simulink model "multiFeedModel"  (R2022a)
settings: Solver=VariableStepAuto  StartTime=0.0  StopTime=168  RelTol=1e-3
model workspace (MAT data in the model file):
  Q_in = [0.12271780758; 0.123470790595; 0.124228393831; 0.124990645638; 0.125757574538; 0.12652920923; 0.127305578587]
libraries: simulink x1
settings Model: Creator=tomok  LastModifiedBy=tomok

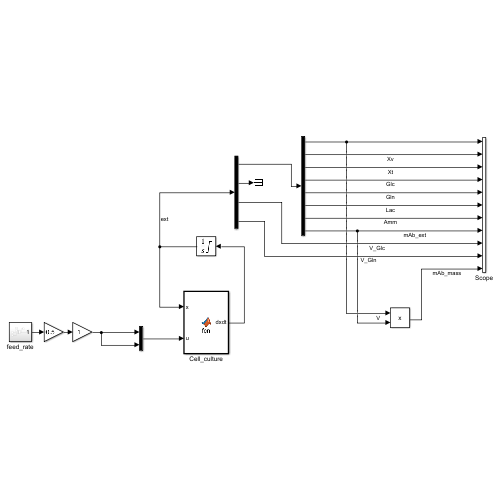
[thumbnail: Simulink's stored preview of the top-level diagram]
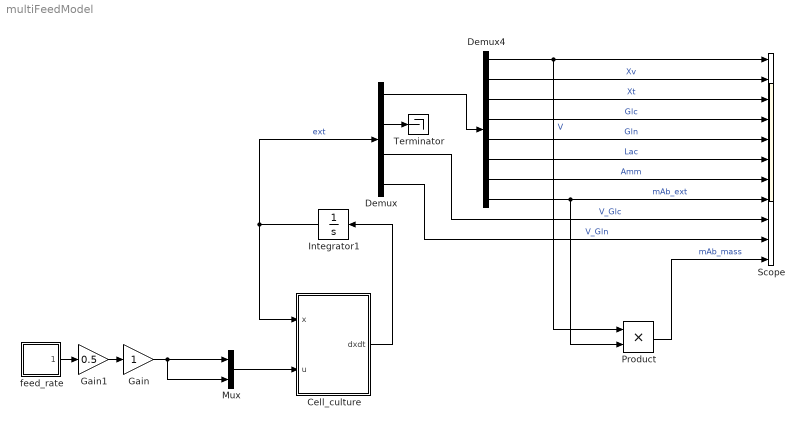
== system multiFeedModel ==
  Cell_culture : MATLAB Function  TreatAsAtomicUnit=on
  Demux : Demux  Outputs=[8,8,1,1]
  Demux4 : Demux  Outputs=8
  Gain : Gain
  Gain1 : Gain  Gain=0.5
  Integrator1 : Integrator  InitialCondition=|  LimitOutput=on  LowerSaturationLimit=0
      | [0.2; 2E+8;
      | 2E+8;
      | 25.1;
      | 5.01;
      | 0;
      | 0;
      | 100; zeros(8,1); 0; 0]
  Mux : Mux  Inputs=2
  Product : Product
  Scope : Scope  NumInputPorts=11
  Terminator : Terminator
  feed_rate : Subsystem
  wires:
  Demux4/1 -> Scope/1, Product/1  "V"
  Product/1 -> Scope/11  "mAb_mass"
  Mux/1 -> Cell_culture/2(u)
  Demux4/5 -> Scope/5  "Gln"
  Demux4/2 -> Scope/2  "Xv"
  Integrator1/1 -> Demux/1, Cell_culture/1(x)  "ext"
  Cell_culture/1(dxdt) -> Integrator1/1
  Demux4/3 -> Scope/3  "Xt"
  Demux4/4 -> Scope/4  "Glc"
  Demux4/7 -> Scope/7  "Amm"
  Demux4/6 -> Scope/6  "Lac"
  Demux4/8 -> Product/2, Scope/8  "mAb_ext"
  feed_rate/1(Out1) -> Gain1/1
  Gain/1 -> Mux/2, Mux/1
  Gain1/1 -> Gain/1
  Demux/1 -> Demux4/1
  Demux/2 -> Terminator/1
  Demux/3 -> Scope/9  "V_Glc"
  Demux/4 -> Scope/10  "V_Gln"

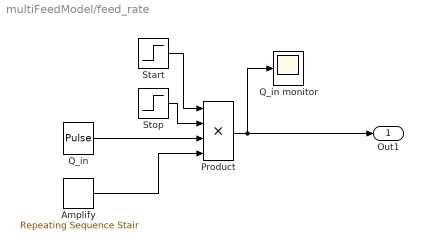
== system multiFeedModel/feed_rate ==
  Amplify : simulink/Sources/Repeating Sequence Stair  OutValues=Q_in  tsamp=24  OutMin=[]  OutMax=[]  OutDataTypeStr=double  OutputDataTypeScalingMode=double  OutDataType=fixdt(0,8)  ConRadixGroup=Best Precision: Vector-wise  OutScaling=2^-12
  Product : Product  Inputs=4
  Q_in : DiscretePulseGenerator  PulseType=Time based  Period=24  PulseWidth=1/24  PhaseDelay=12
  Q_in monitor : Scope
  Start : Step  SampleTime=0
  Stop : Step  Time=169  Before=1  After=0  SampleTime=0
  Out1 : Outport
  wires:
  Stop/1 -> Product/2
  Start/1 -> Product/1
  Product/1 -> Q_in monitor/1, Out1/1
  Q_in/1 -> Product/3
  Amplify/1 -> Product/4

== matlab function multiFeedModel/Cell_culture ==
  data: dxdt output; x input; u input
function dxdt = fcn(x,u)
dxdt = multiFeedStateFcn(x,u);
end
